simulink model "P702_NI_SoftECU"  (R2019a)
settings: Solver=ode1  StartTime=0.0  StopTime=Inf  FixedStep=0.001  RelTol=1e-3  EnableMultiTasking=on
PreLoadFcn:
  | run '.\VeriStand_BlockSet\NIVeriStandAddPaths.m'
undefined symbols (not defined in the file or in its folder): magnitude
libraries: simulink x83, simulink_extras x1
(part 67 of 76)

== system P702_NI_SoftECU/Output/Subsystem2/CAN_Signal/BCM/BCM_Lamp_Stat_0x3C3 ==
  BrkWarnInd_B_Rq : Constant  Value=0
  Brk_Fluid_Lvl_Low : Constant  Value=0
  Courtesy_BSave_Stat : Constant  Value=0
  Courtesy_Delay_Status : Constant  Value=0
  CrnrLghtLeft_Pc_Rq : Constant  Value=0
  CrnrLghtRight_Pc_Rq : Constant  Value=0
  DayRnngLampOn_B_Stat : Constant  Value=0
  DrTgateLck_D_Stat : Constant  Value=0
  Dr_Courtesy_Light_Stat : Constant  Value=0
  HeadLampLoActv_B_Stat : Constant  Value=0
  HeadLampLoFlOn_B_Stat : Constant  Value=0
  HeadLampLoFrOn_B_Stat : Constant  Value=0
  HeadLampLoOut_B_Stat : Constant  Value=0
  HeadLghtHiFdbck_D_Stat : Constant  Value=0
  HeadLghtHiOn_B_Stat : Constant  Value=0
  HeadLghtSwtch_D_Stat : Constant  Value=0
  Headlamp_On_Wrning_Cmd : Constant  Value=0
  HomeSafeLtChime_B_Rq : Constant  Value=0
  Illuminated_Entry_Stat : Constant  Value=0
  ImpactEvntFdbck_D_Stat : Constant  Value=0
  KeyInIgnWarn_B_Cmd : Constant  Value=0
  Park_Brake_Chime_Rqst : Constant  Value=0
  PerimeterAlarmChimeRq : Constant  Value=0
  Perimeter_Alarm_Status : Constant  Value=0
  PrkLght_D_Stat : Constant  Value=0
  PrkLightChime_B_Rq : Constant  Value=0
  PudLampDrv_D_Rq : Constant  Value=0
  PudLampPsngr_D_Rq : Constant  Value=0
  PudLamp_D_Rq : Constant  Value=0
  ReducedGuard_D_Stat : Constant  Value=0
  RvrseLghtOn_B_Stat : Constant  Value=0
  StopLghtOn_B_Stat : Constant  Value=0
  TrnNotInPrkChime_B_Rq : Constant  Value=0
  WndwGlbl_D_Cmd : Constant  Value=0
  WrlssAcsyChrgInhbt_B_Rq : Constant  Value=0
  bus_creator : BusCreator  Inputs=35
  out_port : Outport
  wires:
  bus_creator/1 -> out_port/1  "Subsystem2"
  BrkWarnInd_B_Rq/1 -> bus_creator/1  "BrkWarnInd_B_Rq"
  Brk_Fluid_Lvl_Low/1 -> bus_creator/2  "Brk_Fluid_Lvl_Low"
  Courtesy_BSave_Stat/1 -> bus_creator/3  "Courtesy_BSave_Stat"
  Courtesy_Delay_Status/1 -> bus_creator/4  "Courtesy_Delay_Status"
  CrnrLghtLeft_Pc_Rq/1 -> bus_creator/5  "CrnrLghtLeft_Pc_Rq"
  CrnrLghtRight_Pc_Rq/1 -> bus_creator/6  "CrnrLghtRight_Pc_Rq"
  DayRnngLampOn_B_Stat/1 -> bus_creator/7  "DayRnngLampOn_B_Stat"
  DrTgateLck_D_Stat/1 -> bus_creator/8  "DrTgateLck_D_Stat"
  Dr_Courtesy_Light_Stat/1 -> bus_creator/9  "Dr_Courtesy_Light_Stat"
  HeadLampLoActv_B_Stat/1 -> bus_creator/10  "HeadLampLoActv_B_Stat"
  HeadLampLoFlOn_B_Stat/1 -> bus_creator/11  "HeadLampLoFlOn_B_Stat"
  HeadLampLoFrOn_B_Stat/1 -> bus_creator/12  "HeadLampLoFrOn_B_Stat"
  HeadLampLoOut_B_Stat/1 -> bus_creator/13  "HeadLampLoOut_B_Stat"
  HeadLghtHiFdbck_D_Stat/1 -> bus_creator/14  "HeadLghtHiFdbck_D_Stat"
  HeadLghtHiOn_B_Stat/1 -> bus_creator/15  "HeadLghtHiOn_B_Stat"
  HeadLghtSwtch_D_Stat/1 -> bus_creator/16  "HeadLghtSwtch_D_Stat"
  Headlamp_On_Wrning_Cmd/1 -> bus_creator/17  "Headlamp_On_Wrning_Cmd"
  HomeSafeLtChime_B_Rq/1 -> bus_creator/18  "HomeSafeLtChime_B_Rq"
  Illuminated_Entry_Stat/1 -> bus_creator/19  "Illuminated_Entry_Stat"
  ImpactEvntFdbck_D_Stat/1 -> bus_creator/20  "ImpactEvntFdbck_D_Stat"
  KeyInIgnWarn_B_Cmd/1 -> bus_creator/21  "KeyInIgnWarn_B_Cmd"
  Park_Brake_Chime_Rqst/1 -> bus_creator/22  "Park_Brake_Chime_Rqst"
  PerimeterAlarmChimeRq/1 -> bus_creator/23  "PerimeterAlarmChimeRq"
  Perimeter_Alarm_Status/1 -> bus_creator/24  "Perimeter_Alarm_Status"
  PrkLght_D_Stat/1 -> bus_creator/25  "PrkLght_D_Stat"
  PrkLightChime_B_Rq/1 -> bus_creator/26  "PrkLightChime_B_Rq"
  PudLampDrv_D_Rq/1 -> bus_creator/27  "PudLampDrv_D_Rq"
  PudLampPsngr_D_Rq/1 -> bus_creator/28  "PudLampPsngr_D_Rq"
  PudLamp_D_Rq/1 -> bus_creator/29  "PudLamp_D_Rq"
  ReducedGuard_D_Stat/1 -> bus_creator/30  "ReducedGuard_D_Stat"
  RvrseLghtOn_B_Stat/1 -> bus_creator/31  "RvrseLghtOn_B_Stat"
  StopLghtOn_B_Stat/1 -> bus_creator/32  "StopLghtOn_B_Stat"
  TrnNotInPrkChime_B_Rq/1 -> bus_creator/33  "TrnNotInPrkChime_B_Rq"
  WndwGlbl_D_Cmd/1 -> bus_creator/34  "WndwGlbl_D_Cmd"
  WrlssAcsyChrgInhbt_B_Rq/1 -> bus_creator/35  "WrlssAcsyChrgInhbt_B_Rq"

== system P702_NI_SoftECU/Output/Subsystem2/CAN_Signal/BCM/Battery_Mgmt_24V_0x42E ==
  BattULo24Soc_Pc_Actl : Constant  Value=0
  BattULo24State_D_Qlty : Constant  Value=0
  BattULo24_Ah_DeltaRide : Constant  Value=0
  BattULo24_B_Falt : Constant  Value=0
  BattULo24_I_Actl : Constant  Value=0
  bus_creator : BusCreator  Inputs=5
  out_port : Outport
  wires:
  bus_creator/1 -> out_port/1  "Subsystem2"
  BattULo24_Ah_DeltaRide/1 -> bus_creator/1  "BattULo24_Ah_DeltaRide"
  BattULo24_B_Falt/1 -> bus_creator/2  "BattULo24_B_Falt"
  BattULo24_I_Actl/1 -> bus_creator/3  "BattULo24_I_Actl"
  BattULo24State_D_Qlty/1 -> bus_creator/4  "BattULo24State_D_Qlty"
  BattULo24Soc_Pc_Actl/1 -> bus_creator/5  "BattULo24Soc_Pc_Actl"

== system P702_NI_SoftECU/Output/Subsystem2/CAN_Signal/BCM/Battery_Mgmt_2_0x42C ==
  BattULoChrg_D_Rq : Constant  Value=0
  BattULoSrvc_T_Actl : Constant  Value=0
  Batt_Crit_SoC_B : Constant  Value=0
  Batt_Lo_SoC_B : Constant  Value=0
  ChargeMode : Constant  Value=0
  EngStrtInhbt_B_RqBatt : Constant  Value=0
  IdleSpeedIncrease_El : Constant  Value=0
  PeriodicElLoad_B_Stat : Constant  Value=0
  PwSysULoFalt_D_Stat : Constant  Value=0
  Shed_Drain_Eng_Off_B : Constant  Value=0
  Shed_Feature_Group_ID : Constant  Value=0
  Shed_Level_Req : Constant  Value=0
  Shed_T_Eng_Off_B : Constant  Value=0
  ULoRgenTestMde_B_Rq : Constant  Value=0
  bus_creator : BusCreator  Inputs=14
  out_port : Outport
  wires:
  bus_creator/1 -> out_port/1  "Subsystem2"
  BattULoChrg_D_Rq/1 -> bus_creator/1  "BattULoChrg_D_Rq"
  BattULoSrvc_T_Actl/1 -> bus_creator/2  "BattULoSrvc_T_Actl"
  Batt_Crit_SoC_B/1 -> bus_creator/3  "Batt_Crit_SoC_B"
  Batt_Lo_SoC_B/1 -> bus_creator/4  "Batt_Lo_SoC_B"
  ChargeMode/1 -> bus_creator/5  "ChargeMode"
  EngStrtInhbt_B_RqBatt/1 -> bus_creator/6  "EngStrtInhbt_B_RqBatt"
  IdleSpeedIncrease_El/1 -> bus_creator/7  "IdleSpeedIncrease_El"
  PeriodicElLoad_B_Stat/1 -> bus_creator/8  "PeriodicElLoad_B_Stat"
  PwSysULoFalt_D_Stat/1 -> bus_creator/9  "PwSysULoFalt_D_Stat"
  Shed_Drain_Eng_Off_B/1 -> bus_creator/10  "Shed_Drain_Eng_Off_B"
  Shed_Feature_Group_ID/1 -> bus_creator/11  "Shed_Feature_Group_ID"
  Shed_Level_Req/1 -> bus_creator/12  "Shed_Level_Req"
  Shed_T_Eng_Off_B/1 -> bus_creator/13  "Shed_T_Eng_Off_B"
  ULoRgenTestMde_B_Rq/1 -> bus_creator/14  "ULoRgenTestMde_B_Rq"

== system P702_NI_SoftECU/Output/Subsystem2/CAN_Signal/BCM/Battery_Mgmt_3_0x43C ==
  BSBattQCapAh : Constant  Value=0
  BSBattQDeltaRideAh : Constant  Value=0
  BSBattSOC : Constant  Value=0
  BSFault : Constant  Value=0
  BattULo2_Te_Actl : Constant  Value=0
  BattULoChrg_URate_RqMx : Constant  Value=0
  BattULoChrg_U_RqMn : Constant  Value=0
  BattULoChrg_U_RqMx : Constant  Value=0
  BattULoState_D_Qlty : Constant  Value=0
  bus_creator : BusCreator  Inputs=9
  out_port : Outport
  wires:
  bus_creator/1 -> out_port/1  "Subsystem2"
  BSFault/1 -> bus_creator/1  "BSFault"
  BSBattQDeltaRideAh/1 -> bus_creator/2  "BSBattQDeltaRideAh"
  BSBattSOC/1 -> bus_creator/3  "BSBattSOC"
  BattULo2_Te_Actl/1 -> bus_creator/4  "BattULo2_Te_Actl"
  BSBattQCapAh/1 -> bus_creator/5  "BSBattQCapAh"
  BattULoState_D_Qlty/1 -> bus_creator/6  "BattULoState_D_Qlty"
  BattULoChrg_U_RqMn/1 -> bus_creator/7  "BattULoChrg_U_RqMn"
  BattULoChrg_U_RqMx/1 -> bus_creator/8  "BattULoChrg_U_RqMx"
  BattULoChrg_URate_RqMx/1 -> bus_creator/9  "BattULoChrg_URate_RqMx"

== system P702_NI_SoftECU/Output/Subsystem2/CAN_Signal/BCM/Battery_Mgmt_4_0x42B ==
  BattULoAuxSoc_Pc_Actl : Constant  Value=0
  BattULoAux_B_Falt : Constant  Value=0
  BattULoAux_D_Qlty : Constant  Value=0
  BattULoAux_I_Actl : Constant  Value=0
  BattULoAux_U_Actl : Constant  Value=0
  BattULoCrnkBelt_U_Pred : Constant  Value=0
  BattULoCrnkStrt_U_Pred : Constant  Value=0
  bus_creator : BusCreator  Inputs=7
  out_port : Outport
  wires:
  bus_creator/1 -> out_port/1  "Subsystem2"
  BattULoAux_U_Actl/1 -> bus_creator/1  "BattULoAux_U_Actl"
  BattULoAuxSoc_Pc_Actl/1 -> bus_creator/2  "BattULoAuxSoc_Pc_Actl"
  BattULoAux_B_Falt/1 -> bus_creator/3  "BattULoAux_B_Falt"
  BattULoAux_I_Actl/1 -> bus_creator/4  "BattULoAux_I_Actl"
  BattULoAux_D_Qlty/1 -> bus_creator/5  "BattULoAux_D_Qlty"
  BattULoCrnkBelt_U_Pred/1 -> bus_creator/6  "BattULoCrnkBelt_U_Pred"
  BattULoCrnkStrt_U_Pred/1 -> bus_creator/7  "BattULoCrnkStrt_U_Pred"

== system P702_NI_SoftECU/Output/Subsystem2/CAN_Signal/BCM/BodyInfo_3_0x3B3 ==
  Backlit_LED_Status : Constant  Value=0
  BodySrvcRqd_B_Rq : Constant  Value=0
  CrashEvnt_D_Stat : Constant  Value=0
  Day_Night_Status : Constant  Value=0
  Delay_Accy : Constant  Value=0
  DimmingLvlEvnt_No_Actl : Constant  Value=0
  Dimming_Lvl : Constant  Value=0
  DrStatDrvErrCnt_B_Stat : Constant  Value=0
  DrStatDrv_B_Actl : Constant  Value=0
  DrStatHood_B_Actl : Constant  Value=0
  DrStatInnrTgate_B_Actl : Constant  Value=0
  DrStatPsngr_B_Actl : Constant  Value=0
  DrStatRl_B_Actl : Constant  Value=0
  DrStatRr_B_Actl : Constant  Value=0
  DrStatTgate_B_Actl : Constant  Value=0
  FogLghtFrontOn_B_Stat : Constant  Value=0
  FogLghtRearOn_B_Stat : Constant  Value=0
  FuelPmpInhbt_B_Stat : Constant  Value=0
  IgnKeyType_D_Actl : Constant  Value=0
  Ignition_Status : Constant  Value=0
  Key_In_Ignition_Stat : Constant  Value=0
  LifeCycMde_D_Actl : Constant  Value=0
  Litval : Constant  Value=0
  Parklamp_Status : Constant  Value=0
  PrkBrkActv_B_Actl : Constant  Value=0
  Remote_Start_Status : Constant  Value=0
  TurnLghtLeftOn_B_Stat : Constant  Value=0
  TurnLghtLeft_D_Rq : Constant  Value=0
  TurnLghtRightOn_B_Stat : Constant  Value=0
  TurnLghtRight_D_Rq : Constant  Value=0
  ValetMode_D_Mem : Constant  Value=0
  bus_creator : BusCreator  Inputs=31
  out_port : Outport
  wires:
  bus_creator/1 -> out_port/1  "Subsystem2"
  Ignition_Status/1 -> bus_creator/1  "Ignition_Status"
  Parklamp_Status/1 -> bus_creator/2  "Parklamp_Status"
  FogLghtRearOn_B_Stat/1 -> bus_creator/3  "FogLghtRearOn_B_Stat"
  DrStatTgate_B_Actl/1 -> bus_creator/4  "DrStatTgate_B_Actl"
  Day_Night_Status/1 -> bus_creator/5  "Day_Night_Status"
  Remote_Start_Status/1 -> bus_creator/6  "Remote_Start_Status"
  Key_In_Ignition_Stat/1 -> bus_creator/7  "Key_In_Ignition_Stat"
  BodySrvcRqd_B_Rq/1 -> bus_creator/8  "BodySrvcRqd_B_Rq"
  TurnLghtLeft_D_Rq/1 -> bus_creator/9  "TurnLghtLeft_D_Rq"
  Backlit_LED_Status/1 -> bus_creator/10  "Backlit_LED_Status"
  DrStatDrvErrCnt_B_Stat/1 -> bus_creator/11  "DrStatDrvErrCnt_B_Stat"
  DimmingLvlEvnt_No_Actl/1 -> bus_creator/12  "DimmingLvlEvnt_No_Actl"
  ValetMode_D_Mem/1 -> bus_creator/13  "ValetMode_D_Mem"
  Dimming_Lvl/1 -> bus_creator/14  "Dimming_Lvl"
  IgnKeyType_D_Actl/1 -> bus_creator/15  "IgnKeyType_D_Actl"
  TurnLghtRightOn_B_Stat/1 -> bus_creator/16  "TurnLghtRightOn_B_Stat"
  CrashEvnt_D_Stat/1 -> bus_creator/17  "CrashEvnt_D_Stat"
  FuelPmpInhbt_B_Stat/1 -> bus_creator/18  "FuelPmpInhbt_B_Stat"
  Litval/1 -> bus_creator/19  "Litval"
  PrkBrkActv_B_Actl/1 -> bus_creator/20  "PrkBrkActv_B_Actl"
  TurnLghtLeftOn_B_Stat/1 -> bus_creator/21  "TurnLghtLeftOn_B_Stat"
  LifeCycMde_D_Actl/1 -> bus_creator/22  "LifeCycMde_D_Actl"
  DrStatRr_B_Actl/1 -> bus_creator/23  "DrStatRr_B_Actl"
  DrStatRl_B_Actl/1 -> bus_creator/24  "DrStatRl_B_Actl"
  TurnLghtRight_D_Rq/1 -> bus_creator/25  "TurnLghtRight_D_Rq"
  DrStatDrv_B_Actl/1 -> bus_creator/26  "DrStatDrv_B_Actl"
  DrStatPsngr_B_Actl/1 -> bus_creator/27  "DrStatPsngr_B_Actl"
  DrStatHood_B_Actl/1 -> bus_creator/28  "DrStatHood_B_Actl"
  DrStatInnrTgate_B_Actl/1 -> bus_creator/29  "DrStatInnrTgate_B_Actl"
  Delay_Accy/1 -> bus_creator/30  "Delay_Accy"
  FogLghtFrontOn_B_Stat/1 -> bus_creator/31  "FogLghtFrontOn_B_Stat"

== system P702_NI_SoftECU/Output/Subsystem2/CAN_Signal/BCM/Body_Info_10_0x3BA ==
  GenericSwtch1_No_Actl : Constant  Value=0
  GenericSwtch2_No_Actl : Constant  Value=0
  GenericSwtch3_No_Actl : Constant  Value=0
  bus_creator : BusCreator  Inputs=3
  out_port : Outport
  wires:
  bus_creator/1 -> out_port/1  "Subsystem2"
  GenericSwtch1_No_Actl/1 -> bus_creator/1  "GenericSwtch1_No_Actl"
  GenericSwtch2_No_Actl/1 -> bus_creator/2  "GenericSwtch2_No_Actl"
  GenericSwtch3_No_Actl/1 -> bus_creator/3  "GenericSwtch3_No_Actl"

== system P702_NI_SoftECU/Output/Subsystem2/CAN_Signal/BCM/Body_Info_12_0x26E ==
  FobCtlPssvData_No_Actl : Constant  Value=0
  FobCtlRollCode_No_Stat : Constant  Value=0
  FobCtlType_D_Stat : Constant  Value=0
  bus_creator : BusCreator  Inputs=3
  out_port : Outport
  wires:
  bus_creator/1 -> out_port/1  "Subsystem2"
  FobCtlPssvData_No_Actl/1 -> bus_creator/1  "FobCtlPssvData_No_Actl"
  FobCtlRollCode_No_Stat/1 -> bus_creator/2  "FobCtlRollCode_No_Stat"
  FobCtlType_D_Stat/1 -> bus_creator/3  "FobCtlType_D_Stat"

== system P702_NI_SoftECU/Output/Subsystem2/CAN_Signal/BCM/Body_Info_4_0x242 ==
  BattULo_I_Actl : Constant  Value=0
  BattULo_U_Actl : Constant  Value=0
  BrkTrnShifLck_B_Stat : Constant  Value=0
  DcacElPw_D_Rq : Constant  Value=0
  DriverCrankingReq : Constant  Value=0
  EngOff_T_Actl : Constant  Value=0
  FuelPumpPwr_D_Stat : Constant  Value=0
  PrkLckCtlAvail_T_Stat : Constant  Value=0
  PrkLckCtlMsgTxt_D_Rq : Constant  Value=0
  PrkLckCtlTow_B_Enbl : Constant  Value=0
  PrkLckCtlUnlck_D_Stat : Constant  Value=0
  PrkLckCtl_B_Enbl : Constant  Value=0
  PtLatchActv_B_RqBcm : Constant  Value=0
  ReFuelSwtchStat_D_Actl : Constant  Value=0
  bus_creator : BusCreator  Inputs=15
  immoSecureIdleMode : Constant  Value=0
  out_port : Outport
  wires:
  bus_creator/1 -> out_port/1  "Subsystem2"
  BattULo_I_Actl/1 -> bus_creator/1  "BattULo_I_Actl"
  BattULo_U_Actl/1 -> bus_creator/2  "BattULo_U_Actl"
  BrkTrnShifLck_B_Stat/1 -> bus_creator/3  "BrkTrnShifLck_B_Stat"
  DcacElPw_D_Rq/1 -> bus_creator/4  "DcacElPw_D_Rq"
  DriverCrankingReq/1 -> bus_creator/5  "DriverCrankingReq"
  EngOff_T_Actl/1 -> bus_creator/6  "EngOff_T_Actl"
  FuelPumpPwr_D_Stat/1 -> bus_creator/7  "FuelPumpPwr_D_Stat"
  PrkLckCtlAvail_T_Stat/1 -> bus_creator/8  "PrkLckCtlAvail_T_Stat"
  PrkLckCtlMsgTxt_D_Rq/1 -> bus_creator/9  "PrkLckCtlMsgTxt_D_Rq"
  PrkLckCtlTow_B_Enbl/1 -> bus_creator/10  "PrkLckCtlTow_B_Enbl"
  PrkLckCtlUnlck_D_Stat/1 -> bus_creator/11  "PrkLckCtlUnlck_D_Stat"
  PrkLckCtl_B_Enbl/1 -> bus_creator/12  "PrkLckCtl_B_Enbl"
  PtLatchActv_B_RqBcm/1 -> bus_creator/13  "PtLatchActv_B_RqBcm"
  ReFuelSwtchStat_D_Actl/1 -> bus_creator/14  "ReFuelSwtchStat_D_Actl"
  immoSecureIdleMode/1 -> bus_creator/15  "immoSecureIdleMode"

== system P702_NI_SoftECU/Output/Subsystem2/CAN_Signal/BCM/Body_Info_6_0x38D ==
  DrLatchMsgTxt_D_Rq : Constant  Value=0
  ElPwPoint_D_Rq : Constant  Value=0
  HeadLghtHiPrmsn_D_Stat : Constant  Value=0
  IgnPsswrdDsply_B_Rq : Constant  Value=0
  KeyAdmnTot_No_Cnt : Constant  Value=0
  KeyMykeyTot_No_Cnt : Constant  Value=0
  Keycode_Status : Constant  Value=0
  PEBackupSlot_Stats : Constant  Value=0
  PoliceIdlMde_D_Stat : Constant  Value=0
  PrmtrAlrmEvnt_D_Stat : Constant  Value=0
  PrsnlDevcChrgEnbl_B_Rq : Constant  Value=0
  SecurityMsgTxt_D_Rq : Constant  Value=0
  SteWhlLckMsgTxt_D_Rq : Constant  Value=0
  TracKeyMde_D_Stat : Constant  Value=0
  bus_creator : BusCreator  Inputs=15
  immoMsgTxt_D_Rq : Constant  Value=0
  out_port : Outport
  wires:
  bus_creator/1 -> out_port/1  "Subsystem2"
  KeyAdmnTot_No_Cnt/1 -> bus_creator/1  "KeyAdmnTot_No_Cnt"
  KeyMykeyTot_No_Cnt/1 -> bus_creator/2  "KeyMykeyTot_No_Cnt"
  Keycode_Status/1 -> bus_creator/3  "Keycode_Status"
  PEBackupSlot_Stats/1 -> bus_creator/4  "PEBackupSlot_Stats"
  SteWhlLckMsgTxt_D_Rq/1 -> bus_creator/5  "SteWhlLckMsgTxt_D_Rq"
  immoMsgTxt_D_Rq/1 -> bus_creator/6  "immoMsgTxt_D_Rq"
  PrmtrAlrmEvnt_D_Stat/1 -> bus_creator/7  "PrmtrAlrmEvnt_D_Stat"
  SecurityMsgTxt_D_Rq/1 -> bus_creator/8  "SecurityMsgTxt_D_Rq"
  TracKeyMde_D_Stat/1 -> bus_creator/9  "TracKeyMde_D_Stat"
  DrLatchMsgTxt_D_Rq/1 -> bus_creator/10  "DrLatchMsgTxt_D_Rq"
  PrsnlDevcChrgEnbl_B_Rq/1 -> bus_creator/11  "PrsnlDevcChrgEnbl_B_Rq"
  PoliceIdlMde_D_Stat/1 -> bus_creator/12  "PoliceIdlMde_D_Stat"
  HeadLghtHiPrmsn_D_Stat/1 -> bus_creator/13  "HeadLghtHiPrmsn_D_Stat"
  ElPwPoint_D_Rq/1 -> bus_creator/14  "ElPwPoint_D_Rq"
  IgnPsswrdDsply_B_Rq/1 -> bus_creator/15  "IgnPsswrdDsply_B_Rq"

== system P702_NI_SoftECU/Output/Subsystem2/CAN_Signal/BCM/Body_Info_7_0x3B1 ==
  KeyOffMde_D_Actl : Constant  Value=0
  bus_creator : BusCreator  Inputs=1
  out_port : Outport
  wires:
  bus_creator/1 -> out_port/1  "Subsystem2"
  KeyOffMde_D_Actl/1 -> bus_creator/1  "KeyOffMde_D_Actl"

== system P702_NI_SoftECU/Output/Subsystem2/CAN_Signal/BCM/Body_Info_8_0x3B9 ==
  ChrgCordLck_B_Stat : Constant  Value=0
  ChrgCordResp1_No_Actl : Constant  Value=0
  ChrgCordResp2_No_Actl : Constant  Value=0
  WakeAlarm0_D_Stat : Constant  Value=0
  WakeAlarm1_D_Stat : Constant  Value=0
  WakeAlarm2_D_Stat : Constant  Value=0
  WakeAlarm3_D_Stat : Constant  Value=0
  bus_creator : BusCreator  Inputs=7
  out_port : Outport
  wires:
  bus_creator/1 -> out_port/1  "Subsystem2"
  WakeAlarm0_D_Stat/1 -> bus_creator/1  "WakeAlarm0_D_Stat"
  WakeAlarm1_D_Stat/1 -> bus_creator/2  "WakeAlarm1_D_Stat"
  WakeAlarm2_D_Stat/1 -> bus_creator/3  "WakeAlarm2_D_Stat"
  WakeAlarm3_D_Stat/1 -> bus_creator/4  "WakeAlarm3_D_Stat"
  ChrgCordResp1_No_Actl/1 -> bus_creator/5  "ChrgCordResp1_No_Actl"
  ChrgCordResp2_No_Actl/1 -> bus_creator/6  "ChrgCordResp2_No_Actl"
  ChrgCordLck_B_Stat/1 -> bus_creator/7  "ChrgCordLck_B_Stat"

== system P702_NI_SoftECU/Output/Subsystem2/CAN_Signal/BCM/Body_Info_9_0x3A3 ==
  AdvStrt_D_Stat : Constant  Value=0
  CrnkInhbt_B_Stat : Constant  Value=0
  CrnkInhbt_No_Cnt : Constant  Value=0
  CrnkInhbt_No_Cs : Constant  Value=0
  DrvInCtl_B_Stat : Constant  Value=0
  EngStrtActv_B_Stat : Constant  Value=0
  EngStrt_B_Rq : Constant  Value=0
  IgnPreOffActv_B_Stat : Constant  Value=0
  StrtrMtrCtlDStat_No_Cs : Constant  Value=0
  VehOnSrc_D_Stat : Constant  Value=0
  bus_creator : BusCreator  Inputs=10
  out_port : Outport
  wires:
  bus_creator/1 -> out_port/1  "Subsystem2"
  CrnkInhbt_B_Stat/1 -> bus_creator/1  "CrnkInhbt_B_Stat"
  CrnkInhbt_No_Cnt/1 -> bus_creator/2  "CrnkInhbt_No_Cnt"
  IgnPreOffActv_B_Stat/1 -> bus_creator/3  "IgnPreOffActv_B_Stat"
  DrvInCtl_B_Stat/1 -> bus_creator/4  "DrvInCtl_B_Stat"
  EngStrt_B_Rq/1 -> bus_creator/5  "EngStrt_B_Rq"
  CrnkInhbt_No_Cs/1 -> bus_creator/6  "CrnkInhbt_No_Cs"
  AdvStrt_D_Stat/1 -> bus_creator/7  "AdvStrt_D_Stat"
  VehOnSrc_D_Stat/1 -> bus_creator/8  "VehOnSrc_D_Stat"
  StrtrMtrCtlDStat_No_Cs/1 -> bus_creator/9  "StrtrMtrCtlDStat_No_Cs"
  EngStrtActv_B_Stat/1 -> bus_creator/10  "EngStrtActv_B_Stat"

== system P702_NI_SoftECU/Output/Subsystem2/CAN_Signal/BCM/CMPS_FDM_Info_Status_0x3C7 ==
  CamPDCGuidStat : Constant  Value=0
  CamZoomActiveState : Constant  Value=0
  CamraOvrlDyn_D_Actl : Constant  Value=0
  CamraOvrlStat_D_Actl : Constant  Value=0
  CamraOvrlTow_D_Actl : Constant  Value=0
  CamraViewSplit_D_Actl : Constant  Value=0
  CamraZoomMan_D_Actl : Constant  Value=0
  bus_creator : BusCreator  Inputs=7
  out_port : Outport
  wires:
  bus_creator/1 -> out_port/1  "Subsystem2"
  CamraViewSplit_D_Actl/1 -> bus_creator/1  "CamraViewSplit_D_Actl"
  CamraOvrlDyn_D_Actl/1 -> bus_creator/2  "CamraOvrlDyn_D_Actl"
  CamraZoomMan_D_Actl/1 -> bus_creator/3  "CamraZoomMan_D_Actl"
  CamPDCGuidStat/1 -> bus_creator/4  "CamPDCGuidStat"
  CamZoomActiveState/1 -> bus_creator/5  "CamZoomActiveState"
  CamraOvrlStat_D_Actl/1 -> bus_creator/6  "CamraOvrlStat_D_Actl"
  CamraOvrlTow_D_Actl/1 -> bus_creator/7  "CamraOvrlTow_D_Actl"

== system P702_NI_SoftECU/Output/Subsystem2/CAN_Signal/BCM/CellPhonePassport_Stat_1_0x447 ==
  HeadLghtOn_D_Rq : Constant  Value=0
  KeyProg_No_Actl : Constant  Value=0
  PepsKeyActv_D_Stat : Constant  Value=0
  PepsKeyFound_No_Actl : Constant  Value=0
  Pers1Phone_D_Stat : Constant  Value=0
  Pers2Phone_D_Stat : Constant  Value=0
  Pers3Phone_D_Stat : Constant  Value=0
  Pers4Phone_D_Stat : Constant  Value=0
  RstrtSetting_T_Actl : Constant  Value=0
  Rstrt_T_Actl : Constant  Value=0
  VehLck_D_Dsply : Constant  Value=0
  bus_creator : BusCreator  Inputs=11
  out_port : Outport
  wires:
  bus_creator/1 -> out_port/1  "Subsystem2"
  KeyProg_No_Actl/1 -> bus_creator/1  "KeyProg_No_Actl"
  PepsKeyActv_D_Stat/1 -> bus_creator/2  "PepsKeyActv_D_Stat"
  Rstrt_T_Actl/1 -> bus_creator/3  "Rstrt_T_Actl"
  RstrtSetting_T_Actl/1 -> bus_creator/4  "RstrtSetting_T_Actl"
  PepsKeyFound_No_Actl/1 -> bus_creator/5  "PepsKeyFound_No_Actl"
  HeadLghtOn_D_Rq/1 -> bus_creator/6  "HeadLghtOn_D_Rq"
  VehLck_D_Dsply/1 -> bus_creator/7  "VehLck_D_Dsply"
  Pers1Phone_D_Stat/1 -> bus_creator/8  "Pers1Phone_D_Stat"
  Pers2Phone_D_Stat/1 -> bus_creator/9  "Pers2Phone_D_Stat"
  Pers3Phone_D_Stat/1 -> bus_creator/10  "Pers3Phone_D_Stat"
  Pers4Phone_D_Stat/1 -> bus_creator/11  "Pers4Phone_D_Stat"

== system P702_NI_SoftECU/Output/Subsystem2/CAN_Signal/BCM/GGCC_Config_Mgmt_ID_1_0x40A ==
  VehicleGGCCData : Constant  Value=0
  bus_creator : BusCreator  Inputs=1
  out_port : Outport
  wires:
  bus_creator/1 -> out_port/1  "Subsystem2"
  VehicleGGCCData/1 -> bus_creator/1  "VehicleGGCCData"

== system P702_NI_SoftECU/Output/Subsystem2/CAN_Signal/BCM/GlobalClock_Data_0x84 ==
  GlblClkDay_No_Actl : Constant  Value=0
  GlblClkHr_No_Actl : Constant  Value=0
  GlblClkMnte_No_Actl : Constant  Value=0
  GlblClkScnd_No_Actl : Constant  Value=0
  GlblClkYr_No_Actl : Constant  Value=0
  bus_creator : BusCreator  Inputs=5
  out_port : Outport
  wires:
  bus_creator/1 -> out_port/1  "Subsystem2"
  GlblClkYr_No_Actl/1 -> bus_creator/1  "GlblClkYr_No_Actl"
  GlblClkDay_No_Actl/1 -> bus_creator/2  "GlblClkDay_No_Actl"
  GlblClkMnte_No_Actl/1 -> bus_creator/3  "GlblClkMnte_No_Actl"
  GlblClkScnd_No_Actl/1 -> bus_creator/4  "GlblClkScnd_No_Actl"
  GlblClkHr_No_Actl/1 -> bus_creator/5  "GlblClkHr_No_Actl"

== system P702_NI_SoftECU/Output/Subsystem2/CAN_Signal/BCM/Global_PATS_Control_Info2_0x42 ==
  bus_creator : BusCreator  Inputs=2
  immoControlCmd_T2 : Constant  Value=0
  immoControlData_T2 : Constant  Value=0
  out_port : Outport
  wires:
  bus_creator/1 -> out_port/1  "Subsystem2"
  immoControlCmd_T2/1 -> bus_creator/1  "immoControlCmd_T2"
  immoControlData_T2/1 -> bus_creator/2  "immoControlData_T2"

== system P702_NI_SoftECU/Output/Subsystem2/CAN_Signal/BCM/Global_PATS_Control_Info_0x41 ==
  bus_creator : BusCreator  Inputs=2
  immoControlCmd_T1 : Constant  Value=0
  immoControlData_T1 : Constant  Value=0
  out_port : Outport
  wires:
  bus_creator/1 -> out_port/1  "Subsystem2"
  immoControlCmd_T1/1 -> bus_creator/1  "immoControlCmd_T1"
  immoControlData_T1/1 -> bus_creator/2  "immoControlData_T1"

== system P702_NI_SoftECU/Output/Subsystem2/CAN_Signal/BCM/Locking_Systems_2_0x331 ==
  ChildLckMde_B_Stat : Constant  Value=0
  ChildLck_D_Dsply : Constant  Value=0
  DrTgateExtSwMde_B_Stat : Constant  Value=0
  DrTgateOpen_B_Rq : Constant  Value=0
  FobComm_D_Stat : Constant  Value=0
  Keyfob_Pad_Msg_Count : Constant  Value=0
  L_Pwr_Sliding_Dr_Rqst : Constant  Value=0
  LockInhibit : Constant  Value=0
  Lockmsgtxt_D_Rq : Constant  Value=0
  Power_Decklid_Rqst : Constant  Value=0
  Power_Liftgate_Rqst : Constant  Value=0
  R_Pwr_Sliding_Dr_Rqst : Constant  Value=0
  Remote_Device_Feedback : Constant  Value=0
  RollCodeUnlock : Constant  Value=0
  VehLckInd_D_Rq : Constant  Value=0
  Veh_Lock_EvNum : Constant  Value=0
  Veh_Lock_Requestor : Constant  Value=0
  Veh_Lock_Status : Constant  Value=0
  Veh_Lock_Sub_Id : Constant  Value=0
  WindowLockout_B_Stat : Constant  Value=0
  bus_creator : BusCreator  Inputs=20
  out_port : Outport
  wires:
  bus_creator/1 -> out_port/1  "Subsystem2"
  ChildLck_D_Dsply/1 -> bus_creator/1  "ChildLck_D_Dsply"
  FobComm_D_Stat/1 -> bus_creator/2  "FobComm_D_Stat"
  L_Pwr_Sliding_Dr_Rqst/1 -> bus_creator/3  "L_Pwr_Sliding_Dr_Rqst"
  LockInhibit/1 -> bus_creator/4  "LockInhibit"
  Power_Decklid_Rqst/1 -> bus_creator/5  "Power_Decklid_Rqst"
  Power_Liftgate_Rqst/1 -> bus_creator/6  "Power_Liftgate_Rqst"
  Keyfob_Pad_Msg_Count/1 -> bus_creator/7  "Keyfob_Pad_Msg_Count"
  RollCodeUnlock/1 -> bus_creator/8  "RollCodeUnlock"
  Lockmsgtxt_D_Rq/1 -> bus_creator/9  "Lockmsgtxt_D_Rq"
  R_Pwr_Sliding_Dr_Rqst/1 -> bus_creator/10  "R_Pwr_Sliding_Dr_Rqst"
  WindowLockout_B_Stat/1 -> bus_creator/11  "WindowLockout_B_Stat"
  Veh_Lock_Status/1 -> bus_creator/12  "Veh_Lock_Status"
  DrTgateExtSwMde_B_Stat/1 -> bus_creator/13  "DrTgateExtSwMde_B_Stat"
  Veh_Lock_EvNum/1 -> bus_creator/14  "Veh_Lock_EvNum"
  Veh_Lock_Requestor/1 -> bus_creator/15  "Veh_Lock_Requestor"
  Remote_Device_Feedback/1 -> bus_creator/16  "Remote_Device_Feedback"
  Veh_Lock_Sub_Id/1 -> bus_creator/17  "Veh_Lock_Sub_Id"
  DrTgateOpen_B_Rq/1 -> bus_creator/18  "DrTgateOpen_B_Rq"
  VehLckInd_D_Rq/1 -> bus_creator/19  "VehLckInd_D_Rq"
  ChildLckMde_B_Stat/1 -> bus_creator/20  "ChildLckMde_B_Stat"

== system P702_NI_SoftECU/Output/Subsystem2/CAN_Signal/BCM/PaakRqData1_0x468 ==
  KeyPadCodeProg_D_Stat : Constant  Value=0
  PaakTrgtData_D_Rq : Constant  Value=0
  PaakTrgtPssvData_No_Rq : Constant  Value=0
  PaakTrgtRollCode_No_Rq : Constant  Value=0
  PaakTrgtType_D_Rq : Constant  Value=0
  PaakTrgtZone_D_Rq : Constant  Value=0
  bus_creator : BusCreator  Inputs=6
  out_port : Outport
  wires:
  bus_creator/1 -> out_port/1  "Subsystem2"
  PaakTrgtPssvData_No_Rq/1 -> bus_creator/1  "PaakTrgtPssvData_No_Rq"
  PaakTrgtData_D_Rq/1 -> bus_creator/2  "PaakTrgtData_D_Rq"
  PaakTrgtRollCode_No_Rq/1 -> bus_creator/3  "PaakTrgtRollCode_No_Rq"
  PaakTrgtType_D_Rq/1 -> bus_creator/4  "PaakTrgtType_D_Rq"
  PaakTrgtZone_D_Rq/1 -> bus_creator/5  "PaakTrgtZone_D_Rq"
  KeyPadCodeProg_D_Stat/1 -> bus_creator/6  "KeyPadCodeProg_D_Stat"

== system P702_NI_SoftECU/Output/Subsystem2/CAN_Signal/BCM/PaakRqData2_0x469 ==
  PaakTrgtActvData_No_Rq : Constant  Value=0
  bus_creator : BusCreator  Inputs=1
  out_port : Outport
  wires:
  bus_creator/1 -> out_port/1  "Subsystem2"
  PaakTrgtActvData_No_Rq/1 -> bus_creator/1  "PaakTrgtActvData_No_Rq"

== system P702_NI_SoftECU/Output/Subsystem2/CAN_Signal/BCM/Personality_BCM2_Data_0x3EB ==
  AssocConfirm_D_Actl : Constant  Value=0
  EmPrflKeyAssoc_D_Stat : Constant  Value=0
  EmPrflNo_D_Stat : Constant  Value=0
  Pers1Key_D_Stat : Constant  Value=0
  Pers2Key_D_Stat : Constant  Value=0
  Pers3Key_D_Stat : Constant  Value=0
  Pers4Key_D_Stat : Constant  Value=0
  PersConflict_D_Actl : Constant  Value=0
  PersNoPos_D_Actl : Constant  Value=0
  PersNo_D_Actl : Constant  Value=0
  PersRecallSrc_D_Actl : Constant  Value=0
  PersSetupAccessCtrl : Constant  Value=0
  PersSetupRestr_D_Actl : Constant  Value=0
  PersSetup_No_Actl : Constant  Value=0
  RecallEvent_No_Cnt : Constant  Value=0
  VehKeyActv_D_Stat : Constant  Value=0
  bus_creator : BusCreator  Inputs=16
  out_port : Outport
  wires:
  bus_creator/1 -> out_port/1  "Subsystem2"
  RecallEvent_No_Cnt/1 -> bus_creator/1  "RecallEvent_No_Cnt"
  AssocConfirm_D_Actl/1 -> bus_creator/2  "AssocConfirm_D_Actl"
  Pers1Key_D_Stat/1 -> bus_creator/3  "Pers1Key_D_Stat"
  PersNo_D_Actl/1 -> bus_creator/4  "PersNo_D_Actl"
  PersConflict_D_Actl/1 -> bus_creator/5  "PersConflict_D_Actl"
  PersSetupRestr_D_Actl/1 -> bus_creator/6  "PersSetupRestr_D_Actl"
  PersSetupAccessCtrl/1 -> bus_creator/7  "PersSetupAccessCtrl"
  PersNoPos_D_Actl/1 -> bus_creator/8  "PersNoPos_D_Actl"
  PersSetup_No_Actl/1 -> bus_creator/9  "PersSetup_No_Actl"
  VehKeyActv_D_Stat/1 -> bus_creator/10  "VehKeyActv_D_Stat"
  Pers2Key_D_Stat/1 -> bus_creator/11  "Pers2Key_D_Stat"
  Pers3Key_D_Stat/1 -> bus_creator/12  "Pers3Key_D_Stat"
  EmPrflKeyAssoc_D_Stat/1 -> bus_creator/13  "EmPrflKeyAssoc_D_Stat"
  EmPrflNo_D_Stat/1 -> bus_creator/14  "EmPrflNo_D_Stat"
  Pers4Key_D_Stat/1 -> bus_creator/15  "Pers4Key_D_Stat"
  PersRecallSrc_D_Actl/1 -> bus_creator/16  "PersRecallSrc_D_Actl"

== system P702_NI_SoftECU/Output/Subsystem2/CAN_Signal/BCM/Personality_BCM_Data_0x3E3 ==
  FeatConfigBcmActl : Constant  Value=0
  FeatNoBcm_No_Actl : Constant  Value=0
  FobAssocChime_B_Rq : Constant  Value=0
  LightAmbColor_No_Actl : Constant  Value=0
  LightAmbIntsty_No_Actl : Constant  Value=0
  PersIndexBcm_D_Actl : Constant  Value=0
  bus_creator : BusCreator  Inputs=6
  out_port : Outport
  wires:
  bus_creator/1 -> out_port/1  "Subsystem2"
  FeatConfigBcmActl/1 -> bus_creator/1  "FeatConfigBcmActl"
  FeatNoBcm_No_Actl/1 -> bus_creator/2  "FeatNoBcm_No_Actl"
  PersIndexBcm_D_Actl/1 -> bus_creator/3  "PersIndexBcm_D_Actl"
  FobAssocChime_B_Rq/1 -> bus_creator/4  "FobAssocChime_B_Rq"
  LightAmbColor_No_Actl/1 -> bus_creator/5  "LightAmbColor_No_Actl"
  LightAmbIntsty_No_Actl/1 -> bus_creator/6  "LightAmbIntsty_No_Actl"

== system P702_NI_SoftECU/Output/Subsystem2/CAN_Signal/BCM/Power_Stat_0x456 ==
  RstrnMdulePw_D_Falt : Constant  Value=0
  bus_creator : BusCreator  Inputs=1
  out_port : Outport
  wires:
  bus_creator/1 -> out_port/1  "Subsystem2"
  RstrnMdulePw_D_Falt/1 -> bus_creator/1  "RstrnMdulePw_D_Falt"

== system P702_NI_SoftECU/Output/Subsystem2/CAN_Signal/BCM/RKE_Packet_0x3B6 ==
  Modulation_Ctrl : Constant  Value=0
  RemoteKey_Info_Ctrl : Constant  Value=0
  RemoteKey_Info_Index : Constant  Value=0
  RemoteKey_Info_MaxInd : Constant  Value=0
  RemoteKey_Info_TIC : Constant  Value=0
  TirePress_Filter_Ctrl : Constant  Value=0
  bus_creator : BusCreator  Inputs=6
  out_port : Outport
  wires:
  bus_creator/1 -> out_port/1  "Subsystem2"
  TirePress_Filter_Ctrl/1 -> bus_creator/1  "TirePress_Filter_Ctrl"
  Modulation_Ctrl/1 -> bus_creator/2  "Modulation_Ctrl"
  RemoteKey_Info_Ctrl/1 -> bus_creator/3  "RemoteKey_Info_Ctrl"
  RemoteKey_Info_Index/1 -> bus_creator/4  "RemoteKey_Info_Index"
  RemoteKey_Info_MaxInd/1 -> bus_creator/5  "RemoteKey_Info_MaxInd"
  RemoteKey_Info_TIC/1 -> bus_creator/6  "RemoteKey_Info_TIC"

== system P702_NI_SoftECU/Output/Subsystem2/CAN_Signal/BCM/TPM_Frame_0x3B7 ==
  TirePress_Info_ID : Constant  Value=0
  TirePress_Info_Index : Constant  Value=0
  TirePress_Info_MaxInd : Constant  Value=0
  bus_creator : BusCreator  Inputs=3
  out_port : Outport
  wires:
  bus_creator/1 -> out_port/1  "Subsystem2"
  TirePress_Info_Index/1 -> bus_creator/1  "TirePress_Info_Index"
  TirePress_Info_MaxInd/1 -> bus_creator/2  "TirePress_Info_MaxInd"
  TirePress_Info_ID/1 -> bus_creator/3  "TirePress_Info_ID"

== system P702_NI_SoftECU/Output/Subsystem2/CAN_Signal/BCM/Tire_Pressure_Data_0x3B5 ==
  Tire_Press_LF_Data : Constant  Value=0
  Tire_Press_LR_OLR_Data : Constant  Value=0
  Tire_Press_RF_Data : Constant  Value=0
  Tire_Press_RR_ORR_Data : Constant  Value=0
  bus_creator : BusCreator  Inputs=4
  out_port : Outport
  wires:
  bus_creator/1 -> out_port/1  "Subsystem2"
  Tire_Press_LF_Data/1 -> bus_creator/1  "Tire_Press_LF_Data"
  Tire_Press_RF_Data/1 -> bus_creator/2  "Tire_Press_RF_Data"
  Tire_Press_RR_ORR_Data/1 -> bus_creator/3  "Tire_Press_RR_ORR_Data"
  Tire_Press_LR_OLR_Data/1 -> bus_creator/4  "Tire_Press_LR_OLR_Data"

== system P702_NI_SoftECU/Output/Subsystem2/CAN_Signal/BCM/Tire_Pressure_Data_DRW_0x3B8 ==
  Tire_Press_ILR_Data : Constant  Value=0
  Tire_Press_IRR_Data : Constant  Value=0
  bus_creator : BusCreator  Inputs=2
  out_port : Outport
  wires:
  bus_creator/1 -> out_port/1  "Subsystem2"
  Tire_Press_ILR_Data/1 -> bus_creator/1  "Tire_Press_ILR_Data"
  Tire_Press_IRR_Data/1 -> bus_creator/2  "Tire_Press_IRR_Data"

== system P702_NI_SoftECU/Output/Subsystem2/CAN_Signal/BCM/Tire_Pressure_Stat_0x3B4 ==
  TirePReset_D_Stat : Constant  Value=0
  Tire_Press_ILR_Stat : Constant  Value=0
  Tire_Press_IRR_Stat : Constant  Value=0
  Tire_Press_LF_Stat : Constant  Value=0
  Tire_Press_LR_OLR_Stat : Constant  Value=0
  Tire_Press_Placrd_Frnt : Constant  Value=0
  Tire_Press_Placrd_Rear : Constant  Value=0
  Tire_Press_RF_Stat : Constant  Value=0
  Tire_Press_RR_ORR_Stat : Constant  Value=0
  Tire_Press_System_Stat : Constant  Value=0
  Tire_Press_Telltale : Constant  Value=0
  bus_creator : BusCreator  Inputs=11
  out_port : Outport
  wires:
  bus_creator/1 -> out_port/1  "Subsystem2"
  Tire_Press_System_Stat/1 -> bus_creator/1  "Tire_Press_System_Stat"
  Tire_Press_Telltale/1 -> bus_creator/2  "Tire_Press_Telltale"
  TirePReset_D_Stat/1 -> bus_creator/3  "TirePReset_D_Stat"
  Tire_Press_LF_Stat/1 -> bus_creator/4  "Tire_Press_LF_Stat"
  Tire_Press_RF_Stat/1 -> bus_creator/5  "Tire_Press_RF_Stat"
  Tire_Press_RR_ORR_Stat/1 -> bus_creator/6  "Tire_Press_RR_ORR_Stat"
  Tire_Press_LR_OLR_Stat/1 -> bus_creator/7  "Tire_Press_LR_OLR_Stat"
  Tire_Press_IRR_Stat/1 -> bus_creator/8  "Tire_Press_IRR_Stat"
  Tire_Press_ILR_Stat/1 -> bus_creator/9  "Tire_Press_ILR_Stat"
  Tire_Press_Placrd_Frnt/1 -> bus_creator/10  "Tire_Press_Placrd_Frnt"
  Tire_Press_Placrd_Rear/1 -> bus_creator/11  "Tire_Press_Placrd_Rear"

== system P702_NI_SoftECU/Output/Subsystem2/CAN_Signal/DSMC/CMR_DSMC_AutoSar_NetwrkMgt ==
  CMR_DSMC_AutoSarNMControl : Constant  Value=0
  CMR_DSMC_AutoSarNMNodeId : Constant  Value=0
  CMR_DSMC_AutoSarNMReserve2 : Constant  Value=0
  CMR_DSMC_AutoSarNMReserve3 : Constant  Value=0
  CMR_DSMC_AutoSarNMReserve4 : Constant  Value=0
  CMR_DSMC_AutoSarNMReserved : Constant  Value=0
  CMR_DSMC_GWNMProxY : Constant  Value=0
  CMR_DSMC_GWOnBoardTester : Constant  Value=0
  bus_creator : BusCreator  Inputs=8
  out_port : Outport
  wires:
  bus_creator/1 -> out_port/1  "Subsystem2"
  CMR_DSMC_AutoSarNMControl/1 -> bus_creator/1  "CMR_DSMC_AutoSarNMControl"
  CMR_DSMC_AutoSarNMNodeId/1 -> bus_creator/2  "CMR_DSMC_AutoSarNMNodeId"
  CMR_DSMC_AutoSarNMReserve2/1 -> bus_creator/3  "CMR_DSMC_AutoSarNMReserve2"
  CMR_DSMC_AutoSarNMReserve3/1 -> bus_creator/4  "CMR_DSMC_AutoSarNMReserve3"
  CMR_DSMC_AutoSarNMReserve4/1 -> bus_creator/5  "CMR_DSMC_AutoSarNMReserve4"
  CMR_DSMC_AutoSarNMReserved/1 -> bus_creator/6  "CMR_DSMC_AutoSarNMReserved"
  CMR_DSMC_GWNMProxY/1 -> bus_creator/7  "CMR_DSMC_GWNMProxY"
  CMR_DSMC_GWOnBoardTester/1 -> bus_creator/8  "CMR_DSMC_GWOnBoardTester"

== system P702_NI_SoftECU/Output/Subsystem2/CAN_Signal/DSMC/DrvStatMonData ==
  DrvAlertSt_D_Stat : Constant  Value=0
  DrvAttentZone_D_Stat : Constant  Value=0
  DrvCamDrvIR_D_Stat : Constant  Value=0
  DrvCamPassIR_D_Stat : Constant  Value=0
  DrvCamera_D_Stat : Constant  Value=0
  DrvEngLvlConfid_D_Stat : Constant  Value=0
  DrvEngageLevel_D_Stat : Constant  Value=0
  DrvEngageLevel_No_Cnt : Constant  Value=0
  DrvEngageLevel_No_Cs : Constant  Value=0
  DrvImpLvlConfid_D_Stat : Constant  Value=0
  DrvImpairLvl_D_Stat : Constant  Value=0
  bus_creator : BusCreator  Inputs=11
  out_port : Outport
  wires:
  bus_creator/1 -> out_port/1  "Subsystem2"
  DrvAlertSt_D_Stat/1 -> bus_creator/1  "DrvAlertSt_D_Stat"
  DrvAttentZone_D_Stat/1 -> bus_creator/2  "DrvAttentZone_D_Stat"
  DrvCamDrvIR_D_Stat/1 -> bus_creator/3  "DrvCamDrvIR_D_Stat"
  DrvCamPassIR_D_Stat/1 -> bus_creator/4  "DrvCamPassIR_D_Stat"
  DrvCamera_D_Stat/1 -> bus_creator/5  "DrvCamera_D_Stat"
  DrvEngLvlConfid_D_Stat/1 -> bus_creator/6  "DrvEngLvlConfid_D_Stat"
  DrvEngageLevel_D_Stat/1 -> bus_creator/7  "DrvEngageLevel_D_Stat"
  DrvEngageLevel_No_Cnt/1 -> bus_creator/8  "DrvEngageLevel_No_Cnt"
  DrvEngageLevel_No_Cs/1 -> bus_creator/9  "DrvEngageLevel_No_Cs"
  DrvImpLvlConfid_D_Stat/1 -> bus_creator/10  "DrvImpLvlConfid_D_Stat"
  DrvImpairLvl_D_Stat/1 -> bus_creator/11  "DrvImpairLvl_D_Stat"

== system P702_NI_SoftECU/Output/Subsystem2/CAN_Signal/DSMC/TesterPhysicalResCMR_DSMC ==
  TesterPhysicalResCMR_DSMC : Constant  Value=0
  bus_creator : BusCreator  Inputs=1
  out_port : Outport
  wires:
  bus_creator/1 -> out_port/1  "Subsystem2"
  TesterPhysicalResCMR_DSMC/1 -> bus_creator/1  "TesterPhysicalResCMR_DSMC"

== system P702_NI_SoftECU/Output/Subsystem2/CAN_Signal/ECM_DIESEL PCM PCM_HEV/EngBrakeData_0x165 ==
  AccEngStat_D_Actl : Constant  Value=0
  AccStopMde_D_Rq : Constant  Value=0
  BPedDrvAppl_D_QF : Constant  Value=0
  BpedDrvAppl_D_Actl : Constant  Value=0
  CcMde_D_Actl : Constant  Value=0
  CcOvrrdActv_B_Actl : Constant  Value=0
  CcStat_D_Actl : Constant  Value=0
  CmbbDeny_B_ActlPrpl : Constant  Value=0
  CmbbEngTqMn_B_Actl : Constant  Value=0
  EngAout_N_MnAllw : Constant  Value=0
  PrplTqMnSat_B_Actl : Constant  Value=0
  Veh_V_DsplyCcSet : Constant  Value=0
  bus_creator : BusCreator  Inputs=12
  out_port : Outport
  wires:
  bus_creator/1 -> out_port/1  "Subsystem2"
  CmbbEngTqMn_B_Actl/1 -> bus_creator/1  "CmbbEngTqMn_B_Actl"
  CcOvrrdActv_B_Actl/1 -> bus_creator/2  "CcOvrrdActv_B_Actl"
  BpedDrvAppl_D_Actl/1 -> bus_creator/3  "BpedDrvAppl_D_Actl"
  CmbbDeny_B_ActlPrpl/1 -> bus_creator/4  "CmbbDeny_B_ActlPrpl"
  AccEngStat_D_Actl/1 -> bus_creator/5  "AccEngStat_D_Actl"
  BPedDrvAppl_D_QF/1 -> bus_creator/6  "BPedDrvAppl_D_QF"
  CcMde_D_Actl/1 -> bus_creator/7  "CcMde_D_Actl"
  CcStat_D_Actl/1 -> bus_creator/8  "CcStat_D_Actl"
  Veh_V_DsplyCcSet/1 -> bus_creator/9  "Veh_V_DsplyCcSet"
  AccStopMde_D_Rq/1 -> bus_creator/10  "AccStopMde_D_Rq"
  PrplTqMnSat_B_Actl/1 -> bus_creator/11  "PrplTqMnSat_B_Actl"
  EngAout_N_MnAllw/1 -> bus_creator/12  "EngAout_N_MnAllw"

== system P702_NI_SoftECU/Output/Subsystem2/CAN_Signal/ECM_DIESEL PCM PCM_HEV/EngVehicleSpThrottle2_0x202 ==
  GearRvrse_D_Actl : Constant  Value=0
  StrtrMtrCtlMsgTxt_D2_Rq : Constant  Value=0
  StrtrMtrCtlMsgTxt_D_Rq : Constant  Value=0
  StrtrMtrDlyStrt_B_Stat : Constant  Value=0
  VehVActlEng_D_Qf : Constant  Value=0
  VehVActlEng_No_Cnt : Constant  Value=0
  VehVActlEng_No_Cs : Constant  Value=0
  VehVTrlrAid_B_Avail : Constant  Value=0
  Veh_V_ActlEng : Constant  Value=0
  Veh_V_RqCcSet : Constant  Value=0
  bus_creator : BusCreator  Inputs=10
  out_port : Outport
  wires:
  bus_creator/1 -> out_port/1  "Subsystem2"
  StrtrMtrCtlMsgTxt_D_Rq/1 -> bus_creator/1  "StrtrMtrCtlMsgTxt_D_Rq"
  GearRvrse_D_Actl/1 -> bus_creator/2  "GearRvrse_D_Actl"
  StrtrMtrCtlMsgTxt_D2_Rq/1 -> bus_creator/3  "StrtrMtrCtlMsgTxt_D2_Rq"
  VehVActlEng_No_Cs/1 -> bus_creator/4  "VehVActlEng_No_Cs"
  VehVTrlrAid_B_Avail/1 -> bus_creator/5  "VehVTrlrAid_B_Avail"
  VehVActlEng_No_Cnt/1 -> bus_creator/6  "VehVActlEng_No_Cnt"
  StrtrMtrDlyStrt_B_Stat/1 -> bus_creator/7  "StrtrMtrDlyStrt_B_Stat"
  VehVActlEng_D_Qf/1 -> bus_creator/8  "VehVActlEng_D_Qf"
  Veh_V_RqCcSet/1 -> bus_creator/9  "Veh_V_RqCcSet"
  Veh_V_ActlEng/1 -> bus_creator/10  "Veh_V_ActlEng"

== system P702_NI_SoftECU/Output/Subsystem2/CAN_Signal/ECM_DIESEL PCM PCM_HEV/EngVehicleSpThrottle_0x204 ==
  ApedPosPcActl_D_Qf : Constant  Value=0
  ApedPosPcActl_No_Cnt : Constant  Value=0
  ApedPosPcActl_No_Cs : Constant  Value=0
  ApedPos_PcRate_ActlArb : Constant  Value=0
  ApedPos_Pc_ActlArb : Constant  Value=0
  EngAout3_N_Actl : Constant  Value=0
  EngAoutNActl_D_QF : Constant  Value=0
  EngAout_N_Actl : Constant  Value=0
  bus_creator : BusCreator  Inputs=8
  out_port : Outport
  wires:
  bus_creator/1 -> out_port/1  "Subsystem2"
  ApedPosPcActl_D_Qf/1 -> bus_creator/1  "ApedPosPcActl_D_Qf"
  ApedPosPcActl_No_Cnt/1 -> bus_creator/2  "ApedPosPcActl_No_Cnt"
  ApedPos_Pc_ActlArb/1 -> bus_creator/3  "ApedPos_Pc_ActlArb"
  ApedPos_PcRate_ActlArb/1 -> bus_creator/4  "ApedPos_PcRate_ActlArb"
  EngAoutNActl_D_QF/1 -> bus_creator/5  "EngAoutNActl_D_QF"
  EngAout_N_Actl/1 -> bus_creator/6  "EngAout_N_Actl"
  ApedPosPcActl_No_Cs/1 -> bus_creator/7  "ApedPosPcActl_No_Cs"
  EngAout3_N_Actl/1 -> bus_creator/8  "EngAout3_N_Actl"

== system P702_NI_SoftECU/Output/Subsystem2/CAN_Signal/ECM_DIESEL PCM PCM_HEV/EngineClimateData_0x178 ==
  AirAmbTe_D_Qf : Constant  Value=0
  AirAmb_P_Actl : Constant  Value=0
  AirAmb_Te_Actl : Constant  Value=0
  AirAmb_Te_ActlFilt : Constant  Value=0
  AslChime_B_Rq : Constant  Value=0
  AslIconDsply_D_Rq : Constant  Value=0
  DynoMde_B_Cmd : Constant  Value=0
  EcssLamp_D_RqDsply : Constant  Value=0
  EngAout_Aa_Actl : Constant  Value=0
  GasPrtc_D_RqDsply : Constant  Value=0
  HvacHtrCore2_Te_Actl : Constant  Value=0
  bus_creator : BusCreator  Inputs=11
  out_port : Outport
  wires:
  bus_creator/1 -> out_port/1  "Subsystem2"
  DynoMde_B_Cmd/1 -> bus_creator/1  "DynoMde_B_Cmd"
  AslIconDsply_D_Rq/1 -> bus_creator/2  "AslIconDsply_D_Rq"
  HvacHtrCore2_Te_Actl/1 -> bus_creator/3  "HvacHtrCore2_Te_Actl"
  GasPrtc_D_RqDsply/1 -> bus_creator/4  "GasPrtc_D_RqDsply"
  EcssLamp_D_RqDsply/1 -> bus_creator/5  "EcssLamp_D_RqDsply"
  EngAout_Aa_Actl/1 -> bus_creator/6  "EngAout_Aa_Actl"
  AslChime_B_Rq/1 -> bus_creator/7  "AslChime_B_Rq"
  AirAmbTe_D_Qf/1 -> bus_creator/8  "AirAmbTe_D_Qf"
  AirAmb_Te_Actl/1 -> bus_creator/9  "AirAmb_Te_Actl"
  AirAmb_P_Actl/1 -> bus_creator/10  "AirAmb_P_Actl"
  AirAmb_Te_ActlFilt/1 -> bus_creator/11  "AirAmb_Te_ActlFilt"

== system P702_NI_SoftECU/Output/Subsystem2/CAN_Signal/ECM_DIESEL PCM PCM_HEV/EngineData_6_0x156 ==
  EngClntTe_D_Qf : Constant  Value=0
  EngClnt_Te_Actl : Constant  Value=0
  EngGoutLss_Tq_Est : Constant  Value=0
  EngOil_Te_Actl : Constant  Value=0
  EngOvrhtMitgActv_D_Ind : Constant  Value=0
  bus_creator : BusCreator  Inputs=5
  out_port : Outport
  wires:
  bus_creator/1 -> out_port/1  "Subsystem2"
  EngClnt_Te_Actl/1 -> bus_creator/1  "EngClnt_Te_Actl"
  EngOil_Te_Actl/1 -> bus_creator/2  "EngOil_Te_Actl"
  EngGoutLss_Tq_Est/1 -> bus_creator/3  "EngGoutLss_Tq_Est"
  EngOvrhtMitgActv_D_Ind/1 -> bus_creator/4  "EngOvrhtMitgActv_D_Ind"
  EngClntTe_D_Qf/1 -> bus_creator/5  "EngClntTe_D_Qf"

== system P702_NI_SoftECU/Output/Subsystem2/CAN_Signal/ECM_DIESEL PCM PCM_HEV/EngineData_7_0x179 ==
  AirCondClutch_B_Stats : Constant  Value=0
  AirCondRec_B_Rq : Constant  Value=0
  EngOilLife_Pc_Actl : Constant  Value=0
  EngSrvcRqd_B_Rq : Constant  Value=0
  FuelFillInlet_B_Dsply : Constant  Value=0
  FuelFilterLamp_B_Dsply : Constant  Value=0
  FuelFlw_Vl_Dsply : Constant  Value=0
  HvacAirFullOut_B_Rq : Constant  Value=0
  OdoCount : Constant  Value=0
  TrnKickDown_B_RqDrv : Constant  Value=0
  TrnManShifGear_D_IndDrv : Constant  Value=0
  TrnManShif_D_IndDrv : Constant  Value=0
  bus_creator : BusCreator  Inputs=12
  out_port : Outport
  wires:
  bus_creator/1 -> out_port/1  "Subsystem2"
  TrnManShif_D_IndDrv/1 -> bus_creator/1  "TrnManShif_D_IndDrv"
  HvacAirFullOut_B_Rq/1 -> bus_creator/2  "HvacAirFullOut_B_Rq"
  TrnKickDown_B_RqDrv/1 -> bus_creator/3  "TrnKickDown_B_RqDrv"
  EngSrvcRqd_B_Rq/1 -> bus_creator/4  "EngSrvcRqd_B_Rq"
  EngOilLife_Pc_Actl/1 -> bus_creator/5  "EngOilLife_Pc_Actl"
  FuelFillInlet_B_Dsply/1 -> bus_creator/6  "FuelFillInlet_B_Dsply"
  OdoCount/1 -> bus_creator/7  "OdoCount"
  AirCondRec_B_Rq/1 -> bus_creator/8  "AirCondRec_B_Rq"
  TrnManShifGear_D_IndDrv/1 -> bus_creator/9  "TrnManShifGear_D_IndDrv"
  AirCondClutch_B_Stats/1 -> bus_creator/10  "AirCondClutch_B_Stats"
  FuelFilterLamp_B_Dsply/1 -> bus_creator/11  "FuelFilterLamp_B_Dsply"
  FuelFlw_Vl_Dsply/1 -> bus_creator/12  "FuelFlw_Vl_Dsply"

== system P702_NI_SoftECU/Output/Subsystem2/CAN_Signal/ECM_DIESEL PCM PCM_HEV/Engine_Clutch_Data_0x42F ==
  CluPdlPosPcMeas_D_Qf : Constant  Value=0
  CluPdlPos_Pc_Meas : Constant  Value=0
  CluPdl_PcRate_Actl : Constant  Value=0
  EngAoutIdl_N_Ntrl : Constant  Value=0
  EngAout_N_Dsply : Constant  Value=0
  bus_creator : BusCreator  Inputs=5
  out_port : Outport
  wires:
  bus_creator/1 -> out_port/1  "Subsystem2"
  CluPdl_PcRate_Actl/1 -> bus_creator/1  "CluPdl_PcRate_Actl"
  CluPdlPosPcMeas_D_Qf/1 -> bus_creator/2  "CluPdlPosPcMeas_D_Qf"
  CluPdlPos_Pc_Meas/1 -> bus_creator/3  "CluPdlPos_Pc_Meas"
  EngAoutIdl_N_Ntrl/1 -> bus_creator/4  "EngAoutIdl_N_Ntrl"
  EngAout_N_Dsply/1 -> bus_creator/5  "EngAout_N_Dsply"

== system P702_NI_SoftECU/Output/Subsystem2/CAN_Signal/ECM_DIESEL PCM PCM_HEV/Gear_Shift_by_Wire_3 ==
  GearSelLck_D_Rq : Constant  Value=0
  PrkBrkActv_D_RqTrnGear : Constant  Value=0
  TrnCmdCnt_B_Actl : Constant  Value=0
  TrnCmdState_B_Actl : Constant  Value=0
  TrnDtpCmd_D_Actl : Constant  Value=0
  TrnGearCmd_No_Cnt : Constant  Value=0
  TrnGearCmd_No_Cs : Constant  Value=0
  TrnGearCmd_Pc_ActlPt : Constant  Value=0
  TrnGearMsgTxt_D_Rq : Constant  Value=0
  TrnGearNtmAllow_B_Stat : Constant  Value=0
  TrnGear_D_RqPt : Constant  Value=0
  TrnLvrV_D_Rq : Constant  Value=0
  TrnNtrlTowCmd_D_Actl : Constant  Value=0
  TrnSbwSysHlth_D_Actl : Constant  Value=0
  TrnValidGear_D_Cnfm : Constant  Value=0
  bus_creator : BusCreator  Inputs=15
  out_port : Outport
  wires:
  bus_creator/1 -> out_port/1  "Subsystem2"
  GearSelLck_D_Rq/1 -> bus_creator/1  "GearSelLck_D_Rq"
  PrkBrkActv_D_RqTrnGear/1 -> bus_creator/2  "PrkBrkActv_D_RqTrnGear"
  TrnCmdCnt_B_Actl/1 -> bus_creator/3  "TrnCmdCnt_B_Actl"
  TrnCmdState_B_Actl/1 -> bus_creator/4  "TrnCmdState_B_Actl"
  TrnDtpCmd_D_Actl/1 -> bus_creator/5  "TrnDtpCmd_D_Actl"
  TrnGearCmd_No_Cnt/1 -> bus_creator/6  "TrnGearCmd_No_Cnt"
  TrnGearCmd_No_Cs/1 -> bus_creator/7  "TrnGearCmd_No_Cs"
  TrnGearCmd_Pc_ActlPt/1 -> bus_creator/8  "TrnGearCmd_Pc_ActlPt"
  TrnGearMsgTxt_D_Rq/1 -> bus_creator/9  "TrnGearMsgTxt_D_Rq"
  TrnGearNtmAllow_B_Stat/1 -> bus_creator/10  "TrnGearNtmAllow_B_Stat"
  TrnGear_D_RqPt/1 -> bus_creator/11  "TrnGear_D_RqPt"
  TrnLvrV_D_Rq/1 -> bus_creator/12  "TrnLvrV_D_Rq"
  TrnNtrlTowCmd_D_Actl/1 -> bus_creator/13  "TrnNtrlTowCmd_D_Actl"
  TrnSbwSysHlth_D_Actl/1 -> bus_creator/14  "TrnSbwSysHlth_D_Actl"
  TrnValidGear_D_Cnfm/1 -> bus_creator/15  "TrnValidGear_D_Cnfm"

== system P702_NI_SoftECU/Output/Subsystem2/CAN_Signal/ECM_DIESEL PCM PCM_HEV/Global_PATS_TargetInfo_0x47 ==
  bus_creator : BusCreator  Inputs=3
  immoTarget1Cmd : Constant  Value=0
  immoTarget1Data : Constant  Value=0
  immoTarget1Status : Constant  Value=0
  out_port : Outport
  wires:
  bus_creator/1 -> out_port/1  "Subsystem2"
  immoTarget1Status/1 -> bus_creator/1  "immoTarget1Status"
  immoTarget1Cmd/1 -> bus_creator/2  "immoTarget1Cmd"
  immoTarget1Data/1 -> bus_creator/3  "immoTarget1Data"

== system P702_NI_SoftECU/Output/Subsystem2/CAN_Signal/ECM_DIESEL PCM PCM_HEV/HEV_Powertrain_Data2 ==
  BattTracCnnct_D_Rq : Constant  Value=0
  PrplTqMnRgen_B_Actl : Constant  Value=0
  WhlDirAvgDrv_D_Actl : Constant  Value=0
  bus_creator : BusCreator  Inputs=3
  out_port : Outport
  wires:
  bus_creator/1 -> out_port/1  "Subsystem2"
  BattTracCnnct_D_Rq/1 -> bus_creator/1  "BattTracCnnct_D_Rq"
  PrplTqMnRgen_B_Actl/1 -> bus_creator/2  "PrplTqMnRgen_B_Actl"
  WhlDirAvgDrv_D_Actl/1 -> bus_creator/3  "WhlDirAvgDrv_D_Actl"

== system P702_NI_SoftECU/Output/Subsystem2/CAN_Signal/ECM_DIESEL PCM PCM_HEV/PCM_AutoSar_NetworkMgmt_0x595 ==
  PCM_AutoSarNMControl : Constant  Value=0
  PCM_AutoSarNMNodeId : Constant  Value=0
  PCM_AutoSarNMReserved{1..4} (4 alike) : Constant  Value=0
  PCM_GWNMProxy : Constant  Value=0
  PCM_GWOnBoardTester : Constant  Value=0
  bus_creator : BusCreator  Inputs=8
  out_port : Outport
  wires:
  bus_creator/1 -> out_port/1  "Subsystem2"
  PCM_AutoSarNMNodeId/1 -> bus_creator/1  "PCM_AutoSarNMNodeId"
  PCM_AutoSarNMControl/1 -> bus_creator/2  "PCM_AutoSarNMControl"
  PCM_AutoSarNMReserved1/1 -> bus_creator/3  "PCM_AutoSarNMReserved1"
  PCM_AutoSarNMReserved2/1 -> bus_creator/4  "PCM_AutoSarNMReserved2"
  PCM_GWOnBoardTester/1 -> bus_creator/5  "PCM_GWOnBoardTester"
  PCM_GWNMProxy/1 -> bus_creator/6  "PCM_GWNMProxy"
  PCM_AutoSarNMReserved3/1 -> bus_creator/7  "PCM_AutoSarNMReserved3"
  PCM_AutoSarNMReserved4/1 -> bus_creator/8  "PCM_AutoSarNMReserved4"

== system P702_NI_SoftECU/Output/Subsystem2/CAN_Signal/ECM_DIESEL PCM PCM_HEV/PCM_Rapid_Data_Response_1_0x6A0 ==
  UUDTPCMResponse1 : Constant  Value=0
  bus_creator : BusCreator  Inputs=1
  out_port : Outport
  wires:
  bus_creator/1 -> out_port/1  "Subsystem2"
  UUDTPCMResponse1/1 -> bus_creator/1  "UUDTPCMResponse1"

== system P702_NI_SoftECU/Output/Subsystem2/CAN_Signal/ECM_DIESEL PCM PCM_HEV/PowertrainData_10 ==
  GearEngag_D_Actl : Constant  Value=0
  GearLvr_D_ActlDrv : Constant  Value=0
  GearPos_D_Actl : Constant  Value=0
  GearPos_D_Trg : Constant  Value=0
  GearPos_No_Cnt : Constant  Value=0
  GearPos_No_Cs : Constant  Value=0
  TrnIgnOffDly_T_Rq : Constant  Value=0
  TrnPrkSys_D_Actl : Constant  Value=0
  TrnRng_D_Rq : Constant  Value=0
  bus_creator : BusCreator  Inputs=9
  out_port : Outport
  wires:
  bus_creator/1 -> out_port/1  "Subsystem2"
  GearEngag_D_Actl/1 -> bus_creator/1  "GearEngag_D_Actl"
  GearLvr_D_ActlDrv/1 -> bus_creator/2  "GearLvr_D_ActlDrv"
  GearPos_D_Actl/1 -> bus_creator/3  "GearPos_D_Actl"
  GearPos_D_Trg/1 -> bus_creator/4  "GearPos_D_Trg"
  GearPos_No_Cnt/1 -> bus_creator/5  "GearPos_No_Cnt"
  GearPos_No_Cs/1 -> bus_creator/6  "GearPos_No_Cs"
  TrnIgnOffDly_T_Rq/1 -> bus_creator/7  "TrnIgnOffDly_T_Rq"
  TrnPrkSys_D_Actl/1 -> bus_creator/8  "TrnPrkSys_D_Actl"
  TrnRng_D_Rq/1 -> bus_creator/9  "TrnRng_D_Rq"
